simulink model "gtm_design_baseline2"  (R2023b)
settings: Solver=ode3  StartTime=0.0  StopTime=15  FixedStep=Timestep  MaxStep=.1  RelTol=1e-5
StopFcn:
  | MWSout=grabmws(bdroot);
  | MWSout.lastrun=datestr(now);
values from neighbouring files (symbols this model uses):
  Apqr = sys.a(4:6,4:6)    [runmain.m]    (also in runmain_match.m)
  f0_att = fc_att*Kb_att/Kb_rate    (= 0.125)    [runmain.m]    (also in runmain_match.m = 0.05)
  fc_att = 1/2    (= 0.5)    [runmain.m]    (also in runmain_match.m)
  fc_rate = 1/2    (= 0.5)    [runmain.m]    (also in runmain_match.m = 0)
  fi_att = 1/4    (= 0.25)    [runmain.m]    (also in runmain_match.m)
  fi_rate = 1/4    (= 0.25)    [runmain.m]    (also in runmain_match.m)
  flag_cmd = 0    [runmain.m]    (also in runmain_match.m)
  invBmat = inv(Bmat)    [runmain.m]    (also in runmain_match.m)
  invJ = inv(J)    [runmain.m]    (also in runmain_match.m)
  J = [Ixx 0 -Ixz; 0 Iyy 0; -Ixz 0 Izz]    [runmain.m]    (also in runmain_match.m)
  Kb_att = 1    [runmain.m]    (also in runmain_match.m)
  Kb_rate = 4    [runmain.m]    (also in runmain_match.m = 10)
  mws_designpoint = trimgtm(struct('eas',90,'gamma',0),'elev',1)    [runmain.m]    (also in runmain_match.m)
undefined symbols (not defined in the file or in its folder): Aero, aftfuel, aftfuel_pos, b, bias, Cbar, cg_pos0, cg_shift_gear, DamageCase, DamageModels, DamageOnsetTime, engl_ang, engl_pos, engr_ang, engr_pos, fwdfuel, fwdfuel_pos, Inertia0, Inertia_shift_gear, ref_cg, runway_alt, S, StatesInp, symmetric_aero_on, Timestep, w0, WindDir, WindSpd
libraries: simulink_need_slupdate x28, Servo_Model_lib x18, GTM_aerolib x5, Cross_Product_3D_lib x4, simulink x4, Polyval_lib x3, Euler_to_DCM_lib x2, eomlib x2, engine_T2_lib x2, engine_JetCatP70_lib x2, Vb_Converter_lib x1, sensors_T2_design_lib x1
(part 3 of 3)

== system gtm_design_baseline2/Aircraft Model/Aero/Dynamic Derviatives/Rotary Blended UnDamaged Case/Forced Oscillation ==
  alpha : Inport
  pqr : Inport  Port=2
  Assignment to Lateral : Assignment  IndexMode=Zero-based  IndexOptions=Index vector (dialog)  Indices=[1 3 5]  OutputSizes=[1 1]
  Assignment to Lateral1 : Assignment  IndexMode=Zero-based  IndexOptions=Index vector (dialog)  Indices=[1 3 5]  OutputSizes=[1 1]
  Assignment to Longitudinal : Assignment  IndexMode=Zero-based  IndexOptions=Index vector (dialog)  Indices=[0 2 4]  OutputSizes=[1 1]
  Constant : Constant  Value=zeros(6,1)
  Constant1 : Constant  Value=[0:2]  OutDataTypeStr=uint32
  Constant2 : Constant  Value=[0:2]  OutDataTypeStr=uint32
  Constant3 : Constant  Value=[0:2]  OutDataTypeStr=uint32
  Constant4 : Constant  Value=zeros(6,1)
  Constant5 : Constant  Value=zeros(6,1)
  Demux : Demux  Outputs=3
  PreLookup Index Search : simulink_need_slupdate/PreLookup Index Search  bpData=Aero.dC3_q.alpha  searchMode=Binary Search  cacheBpFlag=on  outputFlag=off  IndexDataType=uint32  extrapMode=Linear Extrapolation  rangeErrorMode=None
  PreLookup Index Search1 : simulink_need_slupdate/PreLookup Index Search  bpData=Aero.dC3_r.rhat  searchMode=Binary Search  cacheBpFlag=on  outputFlag=off  IndexDataType=uint32  extrapMode=Linear Extrapolation  rangeErrorMode=None
  PreLookup Index Search2 : simulink_need_slupdate/PreLookup Index Search  bpData=Aero.dC3_p.phat  searchMode=Binary Search  cacheBpFlag=on  outputFlag=off  IndexDataType=uint32  extrapMode=Linear Extrapolation  rangeErrorMode=None
  PreLookup Index Search3 : simulink_need_slupdate/PreLookup Index Search  bpData=Aero.dC3_q.qhat  searchMode=Binary Search  cacheBpFlag=on  outputFlag=off  IndexDataType=uint32  extrapMode=Linear Extrapolation  rangeErrorMode=None
  PreLookup Index Search4 : simulink_need_slupdate/PreLookup Index Search  bpData=Aero.dC3_p.alpha  searchMode=Binary Search  cacheBpFlag=on  outputFlag=off  IndexDataType=uint32  extrapMode=Linear Extrapolation  rangeErrorMode=None
  PreLookup Index Search5 : simulink_need_slupdate/PreLookup Index Search  bpData=Aero.dC3_r.alpha  searchMode=Binary Search  cacheBpFlag=on  outputFlag=off  IndexDataType=uint32  extrapMode=Linear Extrapolation  rangeErrorMode=None
  pitch : simulink_need_slupdate/Interpolation (n-D) using PreLookup  numDimsPopupSelect=3  explicitNumDims=2  table=Aero.dC3_q.data  interpMethod=Linear  extrapMethod=Linear  rangeErrorMode=None  NumSelectionDims=1
  roll : simulink_need_slupdate/Interpolation (n-D) using PreLookup  numDimsPopupSelect=3  explicitNumDims=2  table=Aero.dC3_p.data  interpMethod=Linear  extrapMethod=Linear  rangeErrorMode=None  NumSelectionDims=1
  yaw : simulink_need_slupdate/Interpolation (n-D) using PreLookup  numDimsPopupSelect=3  explicitNumDims=2  table=Aero.dC3_r.data  interpMethod=Linear  extrapMethod=Linear  rangeErrorMode=None  NumSelectionDims=1
  dC6_p : Outport
  dC6_q : Outport  Port=2
  dC6_r : Outport  Port=3
  wires:
  alpha/1 -> PreLookup Index Search4/1, PreLookup Index Search5/1, PreLookup Index Search/1
  pqr/1 -> Demux/1
  Constant1/1 -> pitch/3
  Demux/2 -> PreLookup Index Search3/1
  Demux/1 -> PreLookup Index Search2/1
  Demux/3 -> PreLookup Index Search1/1
  Constant2/1 -> roll/3
  Constant3/1 -> yaw/3
  Constant/1 -> Assignment to Longitudinal/1
  pitch/1 -> Assignment to Longitudinal/2
  roll/1 -> Assignment to Lateral/2
  Constant4/1 -> Assignment to Lateral/1
  Constant5/1 -> Assignment to Lateral1/1
  yaw/1 -> Assignment to Lateral1/2
  PreLookup Index Search1/1 -> yaw/2
  PreLookup Index Search2/1 -> roll/2
  PreLookup Index Search3/1 -> pitch/2
  Assignment to Lateral/1 -> dC6_p/1
  Assignment to Lateral1/1 -> dC6_r/1
  Assignment to Longitudinal/1 -> dC6_q/1
  PreLookup Index Search/1 -> pitch/1
  PreLookup Index Search4/1 -> roll/1
  PreLookup Index Search5/1 -> yaw/1

== system gtm_design_baseline2/Aircraft Model/Aero/Dynamic Derviatives/Rotary Blended UnDamaged Case/Rotary Balance ==
  alpha : Inport
  beta : Inport  Port=2
  w : Inport  Port=3
  Constant1 : Constant  Value=[0:5]  OutDataTypeStr=uint32
  PreLookup Index Search : simulink_need_slupdate/PreLookup Index Search  bpData=Aero.dC6_w.alpha  searchMode=Binary Search  cacheBpFlag=on  outputFlag=off  IndexDataType=uint32  extrapMode=Linear Extrapolation  rangeErrorMode=None
  PreLookup Index Search1 : simulink_need_slupdate/PreLookup Index Search  bpData=Aero.dC6_w.beta  searchMode=Binary Search  cacheBpFlag=on  outputFlag=off  IndexDataType=uint32  extrapMode=Linear Extrapolation  rangeErrorMode=None
  PreLookup Index Search2 : simulink_need_slupdate/PreLookup Index Search  bpData=Aero.dC6_w.what  searchMode=Binary Search  cacheBpFlag=on  outputFlag=off  IndexDataType=uint32  extrapMode=Linear Extrapolation  rangeErrorMode=None
  TableLookup : simulink_need_slupdate/Interpolation (n-D) using PreLookup  numDimsPopupSelect=4  explicitNumDims=2  table=Aero.dC6_w.data  interpMethod=Linear  extrapMethod=Linear  rangeErrorMode=None  NumSelectionDims=1
  dC6 : Outport
  wires:
  PreLookup Index Search/1 -> TableLookup/1
  beta/1 -> PreLookup Index Search1/1
  alpha/1 -> PreLookup Index Search/1
  TableLookup/1 -> dC6/1
  Constant1/1 -> TableLookup/4
  w/1 -> PreLookup Index Search2/1
  PreLookup Index Search1/1 -> TableLookup/3
  PreLookup Index Search2/1 -> TableLookup/2

== system gtm_design_baseline2/Input Generator/CLAW/Inversion (CV = Rate)/Thrust Model/Left_Engine ==
  Throttle : Inport
  pratio : Inport  Port=2
  tratio : Inport  Port=3
  BypassDynamics : Inport  Port=4
  Jetcat P70 : engine_JetCatP70_lib/Jetcat P70  SystemSampleTime=-1  VariantActivationTime=update diagram  AllowFlexibleInterface=on  Latency=0  AutoFrameSizeCalculation=off
  Thrust (lbf) : Outport
  RPM : Outport  Port=2
  h (slg-ft^2/s) : Outport  Port=3
  Fuel Pump Voltage (V) : Outport  Port=4
  EGT (deg C) : Outport  Port=5
  Fuel Flow (lbs/min) : Outport  Port=6
  wires:
  Throttle/1 -> Jetcat P70/1
  pratio/1 -> Jetcat P70/2
  tratio/1 -> Jetcat P70/3
  BypassDynamics/1 -> Jetcat P70/4
  Jetcat P70/1 -> Thrust (lbf)/1
  Jetcat P70/2 -> RPM/1
  Jetcat P70/3 -> h (slg-ft^2/s)/1
  Jetcat P70/4 -> Fuel Pump Voltage (V)/1
  Jetcat P70/5 -> EGT (deg C)/1
  Jetcat P70/6 -> Fuel Flow (lbs/min)/1

== system gtm_design_baseline2/Input Generator/CLAW/Inversion (CV = Rate)/Thrust Model/Right_Engine ==
  Throttle : Inport
  pratio : Inport  Port=2
  tratio : Inport  Port=3
  BypassDynamics : Inport  Port=4
  Jetcat P70 : engine_JetCatP70_lib/Jetcat P70  SystemSampleTime=-1  VariantActivationTime=update diagram  AllowFlexibleInterface=on  Latency=0  AutoFrameSizeCalculation=off
  Thrust (lbf) : Outport
  RPM : Outport  Port=2
  h (slg-ft^2/s) : Outport  Port=3
  Fuel Pump Voltage (V) : Outport  Port=4
  EGT (deg C) : Outport  Port=5
  Fuel Flow (lbs/min) : Outport  Port=6
  wires:
  Throttle/1 -> Jetcat P70/1
  pratio/1 -> Jetcat P70/2
  tratio/1 -> Jetcat P70/3
  BypassDynamics/1 -> Jetcat P70/4
  Jetcat P70/1 -> Thrust (lbf)/1
  Jetcat P70/2 -> RPM/1
  Jetcat P70/3 -> h (slg-ft^2/s)/1
  Jetcat P70/4 -> Fuel Pump Voltage (V)/1
  Jetcat P70/5 -> EGT (deg C)/1
  Jetcat P70/6 -> Fuel Flow (lbs/min)/1

== matlab function gtm_design_baseline2/Aircraft Model/Engines/Jetcat P70 (Left)/Variable Lag ==
  data: pa input; dp input; tau output
function tau = fcn(pa,dp)
% This block supports an embeddable subset of the MATLAB language.
% See the help menu for details.


if dp >= 0
    if pa >= 50
        tau=1.44;  % time constant = 1.44 sec.
    else
        tau=1.96;  % time constant = 1.96 sec.
    end
else
    %
    %  Power decrease.
    %
    if pa >= 50
        tau=0.85;  % time constant = 0.85 sec.
    else
        tau=1.43;  % time constant = 1.43 sec.
    end
end

== matlab function gtm_design_baseline2/Input Generator/CLAW/Desired Dynamics (CV = Att)/Eulerdot_2_pqr ==
  data: u input; y output; e input
function y = fcn(u,e)
% This block supports the Embedded MATLAB subset.
% See the help menu for details. 

phidot      = u(1);
thetadot    = u(2);
psidot      = u(3);

phi         = e(1);
theta       = e(2);
psi         = e(3);

p = phidot - psidot * sin(theta);
q = thetadot * cos(phi) + psidot * cos(theta) * sin(phi);
r = psidot * cos(theta) * cos(phi) - thetadot * sin(phi);

y = [p;q;r];

== matlab function gtm_design_baseline2/Aircraft Model/Aero/Dynamic Derviatives/Rotary Blended UnDamaged Case/Blending Function ==
  data: alpha input; omega output; beta input; tas input; pqr input; pqr_osc output; B input; Cbar input
function[omega,pqr_osc]= hykal(alpha,beta,tas,pqr,B,Cbar)
% Hybrid Kalviste blending method for use in embedded block in Simulink.
%
% Austin Murch
% Austin.M.Murch@nasa.gov

% Dimension vector outputs.
pqr_osc=zeros(3,1);
omega = 0;
 

% Constants
dtr=pi/180;
knots2ft=1.689;

% Setup variables
pb=pqr(1);
qb=pqr(2);
rb=pqr(3);

alpha = alpha*dtr;
beta = beta*dtr;
omega = 0;

%----Hybrid Kalviste Method----%
whichcase = 0;

%Test for case 1: p_osc = 0
if cos(alpha)*cos(beta) == 0
elseif pb == 0
else
    omega = pb/(cos(alpha)*cos(beta));
    r_osc = rb - omega*sin(alpha)*cos(beta);
    if abs(r_osc) > abs(rb)
    elseif r_osc*rb < 0
    else
        whichcase = 1;
    end
end

%Test for case 2: r_osc = 0
if sin(alpha)*cos(beta) == 0
elseif rb == 0
else
    omega = rb/(sin(alpha)*cos(beta));
    p_osc = pb - omega*cos(alpha)*cos(beta);
    if abs(p_osc) > abs(pb)
    elseif p_osc*pb < 0
    else
        whichcase = 2;
    end
end

%Test for case 3: Omega = 0
if whichcase == 0
    whichcase = 3;
end

 

switch whichcase
    case 1
        omega = pb/(cos(alpha)*cos(beta));
        pqr_osc(1) = 0;        
        pqr_osc(2) = qb - omega*sin(beta);        
        pqr_osc(3) = rb - omega*sin(alpha)*cos(beta);

    case 2
        omega = rb/(sin(alpha)*cos(beta));
        pqr_osc(1) = pb - omega*cos(alpha)*cos(beta);
        pqr_osc(2) = qb - omega*sin(beta);
        pqr_osc(3) = 0;

    case 3
        pqr_osc(1) = pb;
        pqr_osc(2) = qb;
        pqr_osc(3) = rb;
        omega = 0;
end

%-----------------------------------------------% End Hybrid Kalviste

% Scale values for table lookup
b2vt=B/(2*tas*knots2ft);
c2vt=Cbar/(2*tas*knots2ft);
omega=omega*b2vt;
pqr_osc=pqr_osc.*[b2vt;c2vt;b2vt];

== matlab function gtm_design_baseline2/Aircraft Model/Engines/Jetcat P70 (Right)/Variable Lag ==
  data: pa input; dp input; tau output
function tau = fcn(pa,dp)
% This block supports an embeddable subset of the MATLAB language.
% See the help menu for details.


if dp >= 0
    if pa >= 50
        tau=1.44;  % time constant = 1.44 sec.
    else
        tau=1.96;  % time constant = 1.96 sec.
    end
else
    %
    %  Power decrease.
    %
    if pa >= 50
        tau=0.85;  % time constant = 0.85 sec.
    else
        tau=1.43;  % time constant = 1.43 sec.
    end
end

== matlab function gtm_design_baseline2/Aircraft Model/Engines/Engine Alignment ==
  data: T output; Tl input; hl input; Tr input; hr input; TL output; engl_ang parameter; engr_ang parameter; TR output; H output
function [T,TL,TR,H] = eng_angles(Tl,hl,Tr,hr,engl_ang,engr_ang)
% This block supports an embeddable subset of the MATLAB language.
% See the help menu for details. 

% Using the engine alignment angles (set in AC_params_T2.m), compute the 
% off-axis thrust and angular momentum terms.

TL = Tl*[cosd(engl_ang(2))*cosd(engl_ang(3));...
         -sind(engl_ang(3));...
         sind(engl_ang(2))*cosd(engl_ang(3))];
TR = Tr*[cosd(engr_ang(2))*cosd(engr_ang(3));...
         -sind(engr_ang(3));...
         sind(engr_ang(2))*cosd(engr_ang(3))];  
T = TL+TR;

H = hl*[cosd(engl_ang(2))*cosd(engl_ang(3));...
         -sind(engl_ang(3));...
         sind(engl_ang(2))*cosd(engl_ang(3))] + ...
         hr*[cosd(engr_ang(2))*cosd(engr_ang(3));...
         -sind(engr_ang(3));...
         sind(engr_ang(2))*cosd(engr_ang(3))];

== matlab function gtm_design_baseline2/Aircraft Model/LandingGear/LandingForces/Embedded MATLAB Function ==
  data: h input; brakec input; steerc input; Xeom input; F output; GEAR_SPRING parameter; zeta parameter
function F = fcn(h,brakec,steerc,Xeom,GEAR_SPRING,zeta)
% This block supports an embeddable subset of the MATLAB language.
% See the help menu for details. 

BRAKE_DAMPER=5;  %lbf sec/ft
MAX_BRAKES=20;   %lbf

K=GEAR_SPRING*[1;2;1] ;  % lbs*ft/rad; roll, pitch, yaw (Landing Gear Geometry)
GEAR_DAMPER=2*zeta*sqrt(GEAR_SPRING*50); %assume 50 lbs aircraft
C=2*zeta*sqrt(K*50);  %  assume 50 lbs aircraft

uvw=Xeom(1:3);
pqr=Xeom(4:6);
euler=Xeom(10:12);

% Brakes act as damper, with saturation in x, always on in y
% Z force is spring on relative height, damper on vertical velocity
% Torques are spring/damper on euler angles, with psi relative to steering reference
F=[ -1*sign(uvw(1))*max(brakec*BRAKE_DAMPER*abs(uvw(1)),BRAKE_DAMPER);...
    -1*sign(uvw(2))*max(BRAKE_DAMPER*abs(uvw(2)),BRAKE_DAMPER);...
     GEAR_SPRING*h - GEAR_DAMPER*uvw(3);
    -K.*(euler(:)-[0;0;euler(3)]) - C.*pqr(:) + K/2.*[0;0;steerc] ];

== matlab function gtm_design_baseline2/Aircraft Model/AuxiliaryVariables/Atmos76/atmos76 ==
  data: z input; y output; dt input
function y = layer1atm(z,dt)
% Author: Kevin Cunningham          April 20, 1992    
% Modified: Dave Cox                Aug, 14, 2008

y=zeros(6,1);

%dt=0;  % Standard Temp forced.

%    --- constants from 1976 std. atmosphere
r     = 1716.55915670803;
gamma = 1.4;
g     = 32.17405;
re    = 20855531.5;
tsl   = 288.15 * 1.8;
psl   = 2116.22;
hsl   = 0.;
sldens = 0.0023769;                 % atmospheric density at sea level
slpr   = 2116.220;                  % sea level pressure, psf

%---------------------------------------------------------------------
%    conversion from metric lapse rate to english lapse rate
%    meters/0.3048 = ft
%    Kelvin * 1.8 = Rankine
rm2ft = 1000.0/0.3048;
conlapse = 1.8/rm2ft;

%  ---- convert geometric alt. to geopotential alt.
h     = (re*z)/(re+z);
 
%  ---- ensure we are in layer one (based on geopotential alt)
if (h > 11*rm2ft) % 11 km
  %fprintf(1,'Error, atmosphere model out of range %f, Limiting...\n',h);
  h=11*rm2ft;
end
if (h<0)
  %fprintf(1,'Error, atmosphere model out of range %f, Limiting...\n',h);
  h=0;
end

a1     = -6.5*conlapse;
t1     = tsl + a1*(h-hsl);
del1   = (t1/tsl)^(-g/r/a1);
p1     = del1 * psl;

%   ---- apply temperature increment from standard day*/
t1     = t1 + dt;

%   ---- calculate density from eqn. of state w/ corrected temp.*/
rho1   = p1 / (r * t1);
 
%   ---- calculate speed of sound w/ corrected temp.*/
c1     = sqrt(gamma * (r * t1));
 

% Calculate outputs
y(1) = rho1;
y(2) = p1;
y(3) = t1 / 1.8; % output temperature  in Kelvin
y(4) = c1;
y(5) = y(2) / slpr;         % pressure ratio
y(6) = sqrt(y(1)/sldens);   % SQUARE ROOT OF DENSITY RATIO

== matlab function gtm_design_baseline2/Aircraft Model/AuxiliaryVariables/Embedded MATLAB Function ==
  data: omega input; euler input; v input; n_body output; v_dot input
function n_body = accels(omega,euler,v,v_dot)
% Compute body-axis accelerometer measurements.  
% Inputs:
%       omega: body-axis angular rates, [p q r], in rad/sec
%       euler: Euler angles, [phi theta psi], in rad
%           v: body-axis velocities, [u v w], ft/sec
%       v_dot: body-axis accelerations, [udot vdot wdot], ft/sec^2
%
%
% Author: Austin Murch (Austin.M.Murch@nasa.gov)
% Created: 2/19/2008

g0    = 32.174;
phi   = euler(1);
theta = euler(2);

n_body = zeros(3,1);

v_dot = v_dot(:);
omega = omega(:);
v = v(:);

n_body = (v_dot + cross(omega,v))/g0 - [-sin(theta); cos(theta)*sin(phi); cos(theta)*cos(phi)];

n_body = n_body(:);

== matlab function gtm_design_baseline2/Aircraft Model/A//C parameters/Inertia//Mass//CG Shift/fuel cg shift, cg_pos0 ==
  data: fuel_used input; y output; aftfuel parameter; fwdfuel parameter; aftfuel_pos parameter; fwdfuel_pos parameter; w0 parameter; cg_pos0 parameter
function y = fcn(fuel_used,aftfuel,fwdfuel,aftfuel_pos,fwdfuel_pos,w0,cg_pos0)
% This block supports an embeddable subset of the MATLAB language.
% See the help menu for details. 

y = w0.*cg_pos0 - min(aftfuel,fuel_used).*aftfuel_pos - max(0,fuel_used-fwdfuel).*fwdfuel_pos;
